simulink model "manning_test_su_nonlinear"  (R2022b)
settings: Solver=VariableStepAuto  StartTime=0.0  StopTime=5*N  RelTol=1e-3
undefined symbols (not defined in the file): yd_ds
settings Model: Creator=chuan  LastModifiedBy=chuan

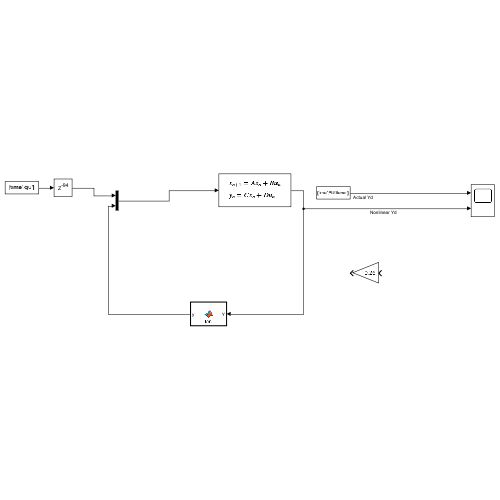
[thumbnail: Simulink's stored preview of the top-level diagram]
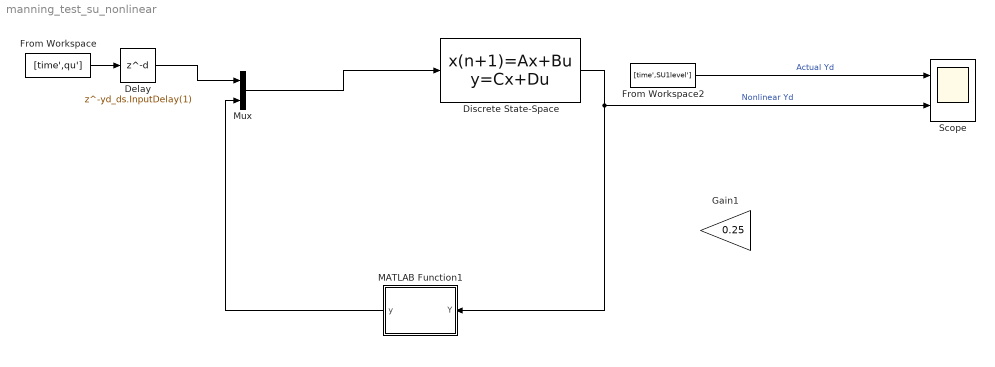
== system manning_test_su_nonlinear ==
  Delay : Delay  DelayLength=yd_ds.InputDelay(1)  InitialCondition=0
  Discrete State-Space : DiscreteStateSpace  A=yd_ds.A  B=yd_ds.B  C=yd_ds.C  D=yd_ds.D  SampleTime=yd_ds.Ts
  From Workspace : FromWorkspace  VariableName=[time',qu']
  From Workspace2 : FromWorkspace  VariableName=[time',SU1level']
  Gain1 : Gain  Gain=0.25
  MATLAB Function1 : MATLAB Function  TreatAsAtomicUnit=on
  Mux : Mux  Inputs=2
  Scope : Scope  NumInputPorts=2
  wires:
  Discrete State-Space/1 -> MATLAB Function1/1(Y), Scope/2  "Nonlinear Yd"
  Mux/1 -> Discrete State-Space/1
  From Workspace2/1 -> Scope/1  "Actual Yd"
  MATLAB Function1/1(y) -> Mux/2
  From Workspace/1 -> Delay/1
  Delay/1 -> Mux/1

== matlab function manning_test_su_nonlinear/MATLAB Function1 ==
  data: Y input; y output
function y = fcn(Y)
Cd = 0.65;
A0 = 36;
g = 9.81;
Z0 = 5.6;
Yfull = 6;
H_star = Z0 + Yfull;

Y = max(Y,0);
H1 = Y + Z0;

if H1 >= H_star
    He = H1 - (Z0 + Yfull/2);
    y = Cd*A0*sqrt(2*g*He);
else
    CwL = (Cd*A0*sqrt(g))/(Yfull);
    y = CwL*(H1-Z0)^(1.5);
end
